simulink model "WT_pitch_actuator"  (R2024a)
settings: Solver=FixedStepAuto  StartTime=0.0  StopTime=10.0  FixedStep=0.001  RelTol=1e-3
settings Model: Creator=ml4  LastModifiedBy=ml4

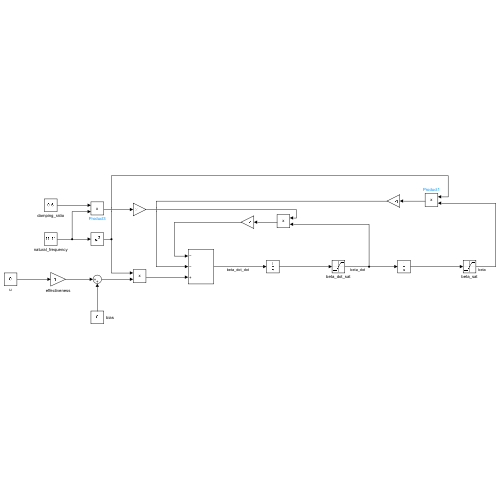
[thumbnail: Simulink's stored preview of the top-level diagram]
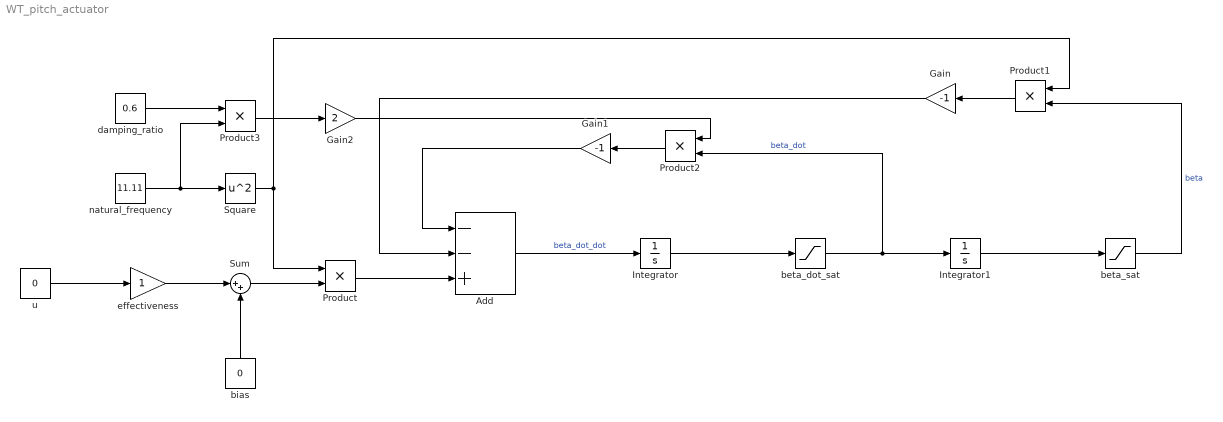
== system WT_pitch_actuator ==
  Add : Sum  Inputs=--+
  Gain : Gain  Gain=-1
  Gain1 : Gain  Gain=-1
  Gain2 : Gain  Gain=2
  Integrator : Integrator
  Integrator1 : Integrator
  Product{,1..3} (4 alike) : Product
  Square : Math  Operator=square
  Sum : Sum  Inputs=|++
  beta_dot_sat : Saturate  UpperLimit=deg2rad(8)  LowerLimit=deg2rad(-8)
  beta_sat : Saturate  UpperLimit=deg2rad(90)  LowerLimit=deg2rad(0)
  bias : Constant  Value=0
  damping_ratio : Constant  Value=0.6
  effectiveness : Gain
  natural_frequency : Constant  Value=11.11
  u : Constant  Value=0
  wires:
  u/1 -> effectiveness/1
  Add/1 -> Integrator/1  "beta_dot_dot"
  Integrator/1 -> beta_dot_sat/1
  beta_dot_sat/1 -> Product2/2, Integrator1/1  "beta_dot"
  Product/1 -> Add/3
  Integrator1/1 -> beta_sat/1
  Product1/1 -> Gain/1
  Product2/1 -> Gain1/1
  beta_sat/1 -> Product1/2  "beta"
  effectiveness/1 -> Sum/1
  Sum/1 -> Product/2
  bias/1 -> Sum/2
  natural_frequency/1 -> Product3/2, Square/1
  Square/1 -> Product1/1, Product/1
  Gain/1 -> Add/2
  Gain1/1 -> Add/1
  damping_ratio/1 -> Product3/1
  Product3/1 -> Gain2/1
  Gain2/1 -> Product2/1
